simulink model "LEDControl"  (R2020b)
settings: Solver=VariableStepAuto  StartTime=0.0  StopTime=1  RelTol=1e-3
libraries: fl_lib x5, nesl_utility x5, ee_lib x2
settings Model: OrderedModelArguments=off  Creator=Miodrag Bolic  LastModifiedBy=bolic
settings DataIOCC: ReturnWorkspaceOutputs=off
settings DebuggingCC: ArithmeticOperatorsInVariantConditions=warning
settings SFSimCC: CustomCodeUndefinedFunction=UseInterfaceOnly

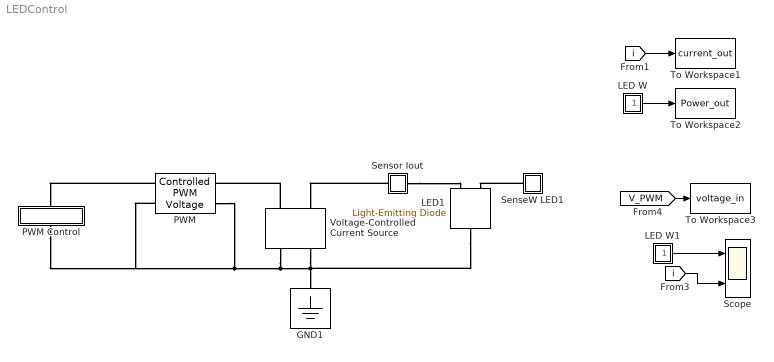
== system LEDControl ==
  GND1 : fl_lib/Electrical/Electrical Elements/Electrical Reference
  LED W : Subsystem
  LED W1 : Subsystem
  LED1 : ee_lib/Sensors & Transducers/Light-Emitting Diode  Gain=0.05 W/A  prmExp=1  I12=[.0017, .003] A  V12=[.9, 1.05] V  IS=5e-5 A  ec=10  RS=0.1 Ohm  Tmeas=25 degC  C_param=1  CJ=20 pF  CJ0=20 pF  VJ=1 V  Mgrad=0.5  Vvec=[.1, 10, 100] V  Cvec=[15, 10, 2] pF  FC=0.5  T_param=1  IS_T2=1.8e-4 A  I1_T2=0.0034 A  V1_T2=1.05 V  Tmeas2=125 degC  EG_param=1  EG=1.11 eV  XTI_param=1  XTI=3  Tdevice=25 degC  i_capacitor_specify=off  i_capacitor_priority=High  i_capacitor=0 A  i_capacitor_nominal_specify=off  i_capacitor_nominal_unit=A  i_capacitor_nominal_value=1  v_capacitor_specify=off  v_capacitor_priority=None  v_capacitor=0 V  v_capacitor_nominal_specify=off  v_capacitor_nominal_unit=V  v_capacitor_nominal_value=1  thermal_network_parameterization=ee.enum.thermalNetworkTopology.cauer  Rth=[0, 10] K/W  Rth_Foster=[4, 6] K/W  thermal_mass_parameterization=ee.enum.thermalNetwork.timeconstant  thermal_mass=[0, 1] J/K  thermal_mass_Foster=[1.5, 3] J/K  thermal_time_constant=[0, 10] s  thermal_time_constant_Foster=[6, 18] s  thermal_mass_initial_temperatures=[25, 25] degC
      settings: SourceProductBaseCode=PS  InternalSimscapePortConfiguration="{\"Bottom\":[],\"Left\":[{\"id\":\"W\",\"label\":\"W\",\"type\":\"output\"},{\"id\":\"p\",\"label\":\"\",\"type\":\"foundation.electrical.electrical\"}],\"Right\":[{\"id\":\"n\",\"label\":\"\",\"type\":\"foundation.electrical.electrical\"}],\"Top\":[]}"
  PWM : ee_lib/Integrated Circuits/Controlled PWM Voltage  F=1000 Hz  TD=0.3 ms  pulse_width_offset=0 s  pulse_min=0 s  Vmin=0 V  Vmax=5 V  Vm=5 V  pwm_or_av=1  event_type=1  sample_time=1e-6 s  u_min=0  u_max=1
  PWM Control : Subsystem
      settings: PortSchema="{\"entries\":[{\"content\":{\"sides\":[{\"content\":{\"connectorIds\":[]},\"type\":\"ConnectorPlacement.EquallySpacedRectSide\",\"uuid\":\"344dc4dd-0ea7-4305-866c-f58732fe9043\"},{\"content\":{\"connectorIds\":[],\"side\":\"RIGHT\"},\"type\":\"ConnectorPlacement.EquallySpacedRectSide\",\"uuid\":\"c7538c69-e6c4-4968-8bfd-16f70b534cb7\"},{\"content\":{\"connectorIds\":[\"LConn1\"],\"side\":\"TOP\"},\"type\":\"ConnectorPlacement.EquallySpacedRectSide\",\"uuid\":\"32dfdc63-f467-46df-8a85-a6c27a880f48\"},{\"content\":{\"connectorIds\":[\"RConn1\"],\"side\":\"BOTTOM\"},\"type\":\"ConnectorPlacement.EquallySpacedRectSide\",\"uuid\":\"d3705a5e-1fac-4960-8372-35c5e51ed885\"},{\"content\":{\"connectorIds\":[],\"side\":\"HIDDEN\"},\"type\":\"ConnectorPlacement.EquallySpacedRectSide\",\"uuid\":\"019f87a5-781f-4ee4-8ec5-add81514c719\"}]},\"type\":\"ConnectorPlacement.EquallySpacedConnector\",\"uuid\":\"070cee4c-c13d-4ce9-8a8d-4ac2ccebb3f2\"}],\"packageUris\":[\"http://schema.mathworks.com/mf0/Connector/R2020b\"],\"version\":\"1.0\"}"
      mask Display:
      | %image('VoltageSource.png'); % Use "Edit Image" on toolstrip to change.
      | disp('Input voltage')
  Scope : Scope  NumInputPorts=2
  SenseW LED1 : Subsystem
  Sensor Iout : Subsystem
      mask Display: disp('i')
  To Workspace1 : ToWorkspace  VariableName=current_out  SaveFormat=Timeseries  SampleTime=-1
  To Workspace2 : ToWorkspace  VariableName=Power_out  SaveFormat=Timeseries  SampleTime=-1
  To Workspace3 : ToWorkspace  VariableName=voltage_in  SaveFormat=Timeseries  SampleTime=-1
  "Voltage-Controlled Current Source " : fl_lib/Electrical/Electrical Sources/Voltage-Controlled Current Source  K=0.005 1/Ohm  v1_specify=off  v1_priority=None  v1=0 V  v1_nominal_specify=off  v1_nominal_unit=V  v1_nominal_value=1  i2_specify=off  i2_priority=None  i2=0 A  i2_nominal_specify=off  i2_nominal_unit=A  i2_nominal_value=1
      settings: SourceProductBaseCode=SS  InternalSimscapePortConfiguration="{\"Bottom\":[],\"Left\":[{\"id\":\"p1\",\"label\":\"+\",\"type\":\"foundation.electrical.electrical\"},{\"id\":\"head\",\"label\":\"\",\"type\":\"foundation.electrical.electrical\"}],\"Right\":[{\"id\":\"n1\",\"label\":\"-\",\"type\":\"foundation.electrical.electrical\"},{\"id\":\"tail\",\"label\":\"\",\"type\":\"foundation.electrical.electrical\"}],\"Top\":[]}"
  wires:
  LED W1/1(W) -> Scope/1
  [i] -> To Workspace1/1
  LED W/1(W) -> To Workspace2/1
  [i] -> Scope/2
  [V_PWM] -> To Workspace3/1
  connections:
  Sensor Iout/LConn1 -- LED1/LConn2
  SenseW LED1/LConn1 -- LED1/LConn1
  Sensor Iout/RConn1 -- "Voltage-Controlled Current Source "/LConn2
  "Voltage-Controlled Current Source "/LConn1 -- PWM/RConn1
  "Voltage-Controlled Current Source "/RConn2 -- PWM/LConn2 -- PWM Control/RConn1 -- PWM/RConn2 -- "Voltage-Controlled Current Source "/RConn1 -- GND1/LConn1 -- LED1/RConn1
  PWM/LConn1 -- PWM Control/LConn1

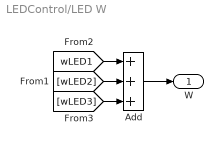
== system LEDControl/LED W ==
  Add : Sum  Inputs=+++
  W : Outport  VectorParamsAs1DForOutWhenUnconnected=off
  wires:
  Add/1 -> W/1
  [wLED1] -> Add/1
  [wLED2] -> Add/2
  [wLED3] -> Add/3

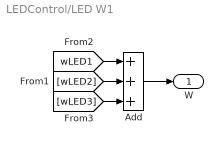
== system LEDControl/LED W1 ==
  Add : Sum  Inputs=+++
  W : Outport  VectorParamsAs1DForOutWhenUnconnected=off
  wires:
  Add/1 -> W/1
  [wLED1] -> Add/1
  [wLED2] -> Add/2
  [wLED3] -> Add/3

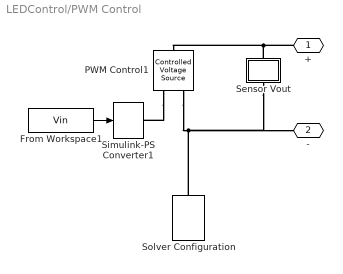
== system LEDControl/PWM Control ==
  From Workspace1 : FromWorkspace  VariableName=Vin  SampleTime=0.0001  OutputAfterFinalValue=Setting to zero
  PWM Control1 : fl_lib/Electrical/Electrical Sources/Controlled Voltage Source
  Sensor Vout : Subsystem
      settings: PortSchema="{\"entries\":[{\"content\":{\"sides\":[{\"content\":{\"connectorIds\":[]},\"type\":\"ConnectorPlacement.EquallySpacedRectSide\",\"uuid\":\"b1bcf9f4-15a1-4e38-81ab-67de1458f8d1\"},{\"content\":{\"connectorIds\":[],\"side\":\"RIGHT\"},\"type\":\"ConnectorPlacement.EquallySpacedRectSide\",\"uuid\":\"ecda133a-47d8-41fe-b4fd-353e3809ddf6\"},{\"content\":{\"connectorIds\":[\"LConn1\"],\"side\":\"TOP\"},\"type\":\"ConnectorPlacement.EquallySpacedRectSide\",\"uuid\":\"d852e0b5-4696-49c9-84f3-2cf03f3856d9\"},{\"content\":{\"connectorIds\":[\"RConn1\"],\"side\":\"BOTTOM\"},\"type\":\"ConnectorPlacement.EquallySpacedRectSide\",\"uuid\":\"f379564a-bafe-4cf9-8574-9ef4aba5b963\"},{\"content\":{\"connectorIds\":[],\"side\":\"HIDDEN\"},\"type\":\"ConnectorPlacement.EquallySpacedRectSide\",\"uuid\":\"a82549ad-b0b3-4bc9-b302-ce3c9536ea9c\"}]},\"type\":\"ConnectorPlacement.EquallySpacedConnector\",\"uuid\":\"d2ad3a19-6b9d-4a5d-9a4f-eec5a8e47e63\"}],\"packageUris\":[\"http://schema.mathworks.com/mf0/Connector/R2020b\"],\"version\":\"1.0\"}"
      mask Display: disp('Vo')
  Simulink-PS Converter1 : nesl_utility/Simulink-PS Converter  PhysicalDomain=network_engine_domain  SubClassName=ps_input  LeftPortType=input  RightPortType=output  PseudoPeriodic=off  Frequencies=[]  NoiseDistribution=none  NoiseParameters=[]  Unit=1  AffineConversion=off  FilteringAndDerivatives=zero  SimscapeFilterOrder=1  InputFilterTimeConstant=0.001  UdotUserProvided=1
  Solver Configuration : nesl_utility/Solver Configuration  PhysicalDomain=network_engine_domain  SubClassName=solver  LeftPortType=input  RightPortType=generic  Tones=[]  Harmonics=[]  SimulateNoise=off  Profile=off  UseLocalSampling=off  EnableSwitchedLinearOptims=on  FrequencyDomain=off  UseCCode=off  RelTol=0.001  AbsTol=1e-06  MinStep=1e-09  ToWorkspace=off  RevertToSquareIcSolve=off  NumHomotopyIterations=100  PhasorMode=off  PhasorModeNumHarmonics=1  DoDC=off  ResidualTolerance=1e-09  UseLocalSolver=off  LocalSolverChoice=NE_BACKWARD_EULER_ADVANCER  LocalSolverSampleTime=0.001  DoFixedCost=off  MaxNonlinIter=3  MaxModeIter=2  ComputeImpulses=off  ImpulseIterations=2  LinearAlgebra=Sparse  EquationFormulation=NE_TIME_EF  DelaysMemoryBudget=1024  AutomaticFiltering=on  FilteringTimeConstant=0.001  PartitionStorageMethod=AS_NEEDED  PartitionMemoryBudget=1024  PartitionMethod=FAST
  + : PMIOPort  Side=Left
  - : PMIOPort  Port=2  Side=Right
  wires:
  From Workspace1/1 -> Simulink-PS Converter1/1
  connections:
  PWM Control1/RConn1 -- Simulink-PS Converter1/RConn1
  Solver Configuration/RConn1 -- Sensor Vout/RConn1 -- -/RConn1 -- PWM Control1/RConn2
  Sensor Vout/LConn1 -- PWM Control1/LConn1 -- +/RConn1

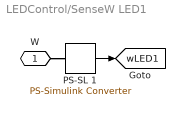
== system LEDControl/SenseW LED1 ==
  PS-SL 1 : nesl_utility/PS-Simulink Converter  PhysicalDomain=network_engine_domain  SubClassName=ps_output  LeftPortType=input  RightPortType=output  PseudoPeriodic=off  Frequencies=[]  Unit=W  AffineConversion=off
  W : PMIOPort  Side=Left
  tag scope: wLED1=global
  wires:
  PS-SL 1/1 -> [wLED1]
  connections:
  W/RConn1 -- PS-SL 1/LConn1

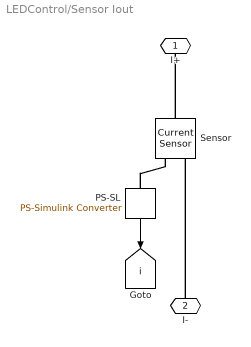
== system LEDControl/Sensor Iout ==
  PS-SL : nesl_utility/PS-Simulink Converter  PhysicalDomain=network_engine_domain  SubClassName=ps_output  LeftPortType=input  RightPortType=output  PseudoPeriodic=off  Frequencies=[]  Unit=1  AffineConversion=off
  Sensor : fl_lib/Electrical/Electrical Sensors/Current Sensor
      settings: SourceProductName=Foundation Library
  I+ : PMIOPort  Side=Right
  I- : PMIOPort  Port=2  Side=Left
  tag scope: i=global
  wires:
  PS-SL/1 -> [i]
  connections:
  PS-SL/LConn1 -- Sensor/RConn1
  Sensor/LConn1 -- I+/RConn1
  I-/RConn1 -- Sensor/RConn2

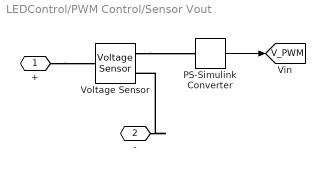
== system LEDControl/PWM Control/Sensor Vout ==
  PS-Simulink Converter : nesl_utility/PS-Simulink Converter  PhysicalDomain=network_engine_domain  SubClassName=ps_output  LeftPortType=input  RightPortType=output  PseudoPeriodic=off  Frequencies=[]  Unit=1  AffineConversion=off
      settings: SourceProductName=Utilities
  Voltage Sensor : fl_lib/Electrical/Electrical Sensors/Voltage Sensor
      settings: SourceProductName=Foundation Library
  + : PMIOPort  Side=Left
  - : PMIOPort  Port=2  Side=Right
  tag scope: V_PWM=global
  wires:
  PS-Simulink Converter/1 -> [V_PWM]
  connections:
  -/RConn1 -- Voltage Sensor/RConn2
  Voltage Sensor/RConn1 -- PS-Simulink Converter/LConn1
  +/RConn1 -- Voltage Sensor/LConn1
